simulink model "SiEngineController"  (R2024a)
settings: configuration reference "EngFixed10ms" (kept outside this file)
undefined symbols (not defined in the file): CtrlEcuTs, PlntEngAfrStoich
libraries: autolibengctrlr x1
settings Model: DataDictionary=VirtualDynoTemplate.sldd  ModifiedByFormat=The MathWorks, Inc.  Creator=The MathWorks, Inc.  LastModifiedBy=The MathWorks, Inc.
settings ConfigSetRef: SourceName=EngFixed10ms

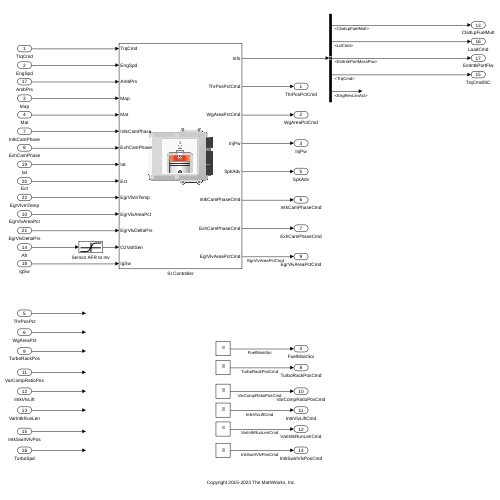
[thumbnail: Simulink's stored preview of the top-level diagram]
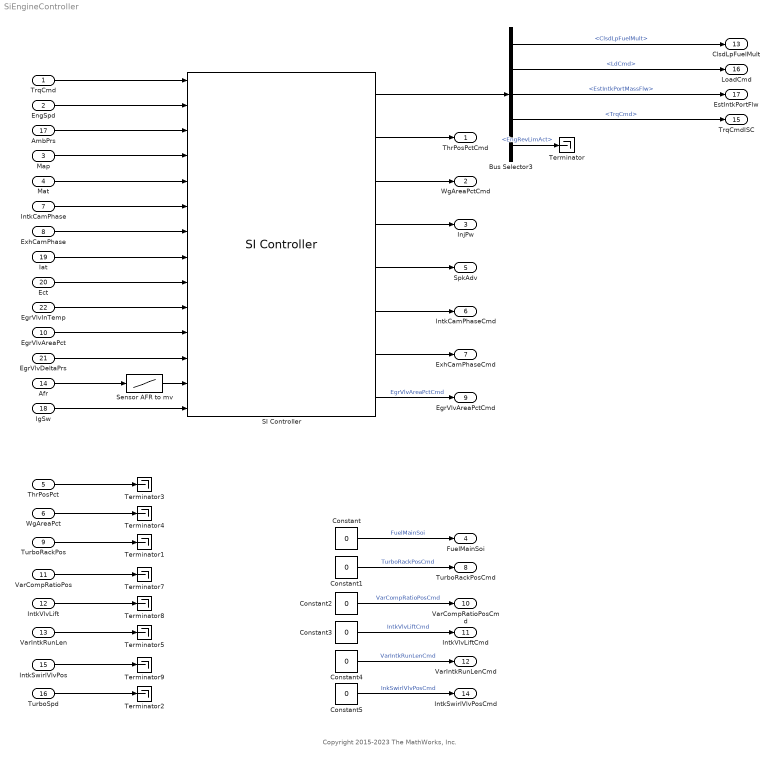
== system SiEngineController ==
  note: Copyright 2015-2023 The MathWorks, Inc.
  TrqCmd : Inport  OutDataTypeStr=double  Unit=N*m  PortDimensions=1
  EngSpd : Inport  Port=2  OutDataTypeStr=double  Unit=rpm  PortDimensions=1
  Map : Inport  Port=3  OutDataTypeStr=double  Unit=Pa  PortDimensions=1
  Mat : Inport  Port=4  OutDataTypeStr=double  Unit=K  PortDimensions=1
  ThrPosPct : Inport  Port=5  OutDataTypeStr=double  Unit=%  PortDimensions=1
  WgAreaPct : Inport  Port=6  OutDataTypeStr=double  Unit=%  PortDimensions=1
  IntkCamPhase : Inport  Port=7  OutDataTypeStr=double  Unit=deg  PortDimensions=1
  ExhCamPhase : Inport  Port=8  OutDataTypeStr=double  Unit=deg  PortDimensions=1
  TurboRackPos : Inport  Port=9  OutDataTypeStr=double  Unit=1  PortDimensions=1
  EgrVlvAreaPct : Inport  Port=10  OutDataTypeStr=double  Unit=%  PortDimensions=1
  VarCompRatioPos : Inport  Port=11  OutDataTypeStr=double  PortDimensions=1
  IntkVlvLift : Inport  Port=12  OutDataTypeStr=double  PortDimensions=1
  VarIntkRunLen : Inport  Port=13  OutDataTypeStr=double  PortDimensions=1
  Afr : Inport  Port=14  OutDataTypeStr=double  Unit=1  PortDimensions=1
  IntkSwirlVlvPos : Inport  Port=15  OutDataTypeStr=double  PortDimensions=1
  TurboSpd : Inport  Port=16  OutDataTypeStr=double  Unit=rpm  PortDimensions=1
  AmbPrs : Inport  Port=17  OutDataTypeStr=double  Unit=Pa  PortDimensions=1
  IgSw : Inport  Port=18  OutDataTypeStr=boolean  PortDimensions=1
  Iat : Inport  Port=19  OutDataTypeStr=double  Unit=K  PortDimensions=1
  Ect : Inport  Port=20  OutDataTypeStr=double  Unit=K  PortDimensions=1
  EgrVlvDeltaPrs : Inport  Port=21  OutDataTypeStr=double  Unit=Pa  PortDimensions=1
  EgrVlvInTemp : Inport  Port=22  OutDataTypeStr=double  Unit=K  PortDimensions=1
  Bus Selector3 : BusSelector  OutputSignals=ClsdLpFuelMult,LdCmd,EstIntkPortMassFlw,TrqCmd,EngRevLimAct
  Constant{,1..5} (6 alike) : Constant  Value=0  SampleTime=-1
  SI Controller : autolibengctrlr/SI Controller  AirEstOptionPopup=Dual Variable Cam Phasing  TrqEstOptionPopup=Torque Structure  f_lcmd=CtrlEcuLCmd  f_lcmd_tq_bpt=CtrlEcuLCmdTqBpt  f_lcmd_n_bpt=CtrlEcuLCmdSpdBpt  f_tap=CtrlEcuTap  f_tap_ld_bpt=CtrlEcuTapLBpt  f_tap_n_bpt=CtrlEcuTapNBpt  f_tpp=CtrlEcuTpp  f_tpp_tap_bpt=CtrlEcuTppTapBpt  f_wap=CtrlEcuWap  f_wap_ld_bpt=CtrlEcuWapLBpt  f_wap_n_bpt=CtrlEcuWapNBpt  f_icp=CtrlEcuIcp  f_ecp=CtrlEcuEcp  f_cp_ld_bpt=CtrlEcuCpLBpt  f_cp_n_bpt=CtrlEcuCpNBpt  f_egrpct_cmd=CtrlEcuEgrCmd  f_egrpct_ld_bpt=CtrlEcuEgrCmdLBpt  f_egrpct_n_bpt=CtrlEcuEgrCmdNBpt  f_egr_areapct_cmd=CtrlEcuEgrAreaCmd  f_egr_max_stdflow=CtrlEcuEgrMaxStdFlw  f_egr_areapct_nrmlzdflow_bpt=CtrlEcuEgrAreaNrmFlwBpt  f_egr_areapct_pr_bpt=CtrlEcuEgrAreaPrBpt  LambdaCmdOvrd=off  Sinj=PlntEngSinj  Nmin=1  afr_stoich=PlntEngAfrStoich  f_lamcmd=CtrlEcuLamCmd  f_lamcmd_ld_bpt=CtrlEcuLamCmdLBpt  f_lamcmd_n_bpt=CtrlEcuLamCmdNBpt  f_startup_lambda_delta=CtrlEcuStUpLamDelta  f_startup_lambda_delta_timecnst=CtrlEcuStUpLamDeltaTimeC  f_startup_ect_bpt=CtrlEcuStUpEctBpt  ClsdLpFuelEn=off  OpenLpDitherEn=off  LambdaDitherAmp=0.03  LambdaDitherFrq=0.75  ClsdLpFuelPGain=0.005  ClsdLpFuelIGain=0.05  ClsdLpFuelIntgLmt=0.2  O2ResetStoichVoltSen=2500  O2ResetMinVoltSen=0  O2ResetMaxVoltSen=5000  O2LearnUpdatePerSen=4  O2AmpMinVoltSen=250  O2ReadyVoltSen=1150  O2NotReadyVoltSen=1950  f_sa=CtrlEcuSa  f_sa_ld_bpt=CtrlEcuSaLBpt  f_sa_n_bpt=CtrlEcuSaNBpt  N_idle=CtrlEcuNidle  Trq_idlecmd_enable=1  Trq_idlecmd_max=50  Kp_idle=0.02  Ki_idle=0.01  EngRevLim=CtrlEcuRevLim  CrankSpeed=CtrlEcuCrkSpd  ESSEnable=on  ESSExternalPortEnable=off  EngStopTime=CtrlEcuStopTime  CatLightOffTime=CtrlEcuCatLOff  Ts=CtrlEcuTs  NCyl=PlntEngNCyl  Cps=PlntEngCps  Vd=PlntEngVd  Rair=EnvRair  Pstd=EnvAbsPrs  Tstd=EnvAirTemp  f_nv=PlntEngNv  f_nv_prs_bpt=PlntEngNvPrBpt  f_nv_n_bpt=PlntEngNvSpdBpt  f_vivc=PlntEngVivc  f_tm_corr_n_bpt=PlntEngTmCorrNBpt  f_vivc_icp_bpt=PlntEngVivcBpt  f_tm_corr=PlntEngTmCorr  f_tm_corr_nd_bpt=PlntEngTmCorrNdBpt  f_mdot_intk=CtrlEngMdotIntk  f_mdot_intk_ecp_bpt=PlntEngMdotIntkEcpBpt  f_mdot_trpd_bpt=PlntEngMdotTrpdBpt  f_mdot_air_corr=PlntEngMdotAirCorr  f_mdot_air_corr_ld_bpt=PlntEngMdotAirCorrLdBpt  f_mdot_air_n_bpt=PlntEngMdotAirCorrNBpt  tau_egr=CtrlEcuEgrTau  f_intksys_stdflow_pr=CtrlEcuInkStdFlwPr  f_intksys_stdflow_bpt=CtrlEcuInkStdFlwBpt  f_egr_stdflow=CtrlEcuEgrStdFlw  f_egr_stdflow_pr_bpt=CtrlEcuEgrStdFlwPrBpt  f_egr_stdflow_egrap_bpt=CtrlEcuEgrStdFlwEgrApBpt  f_tq_nl=PlntEngTqTbl  f_tq_nl_l_bpt=PlntEngTqTblLBpt  f_tq_nl_n_bpt=PlntEngTqTblNBpt  f_tq_inr=CtrlEngInTrqMap  f_tq_fric=CtrlEngTqFric  f_fric_temp_mod=PlntEngFricTMod  f_fric_temp_bpt=PlntEngFricTBpt  f_tq_pump=CtrlEngTqPump  f_sa_opt=CtrlEngSAOpt  f_tq_inr_l_bpt=CtrlEngInTrqLdBpt  f_tq_inr_n_bpt=CtrlEngInTrqSpdBpt  f_m_sa=PlntEngMSa  f_del_sa_bpt=PlntEngDelSaBpt  f_m_lam=PlntEngMLam  f_m_lam_bpt=PlntEngMLamBpt  f_t_exh=PlntEngTexh  f_t_exh_l_bpt=PlntEngTexhLBpt  f_t_exh_n_bpt=PlntEngTexhNBpt
  Sensor AFR to mv : Lookup  InputValues="PlntEngAfrStoich+[-0.1460         0    0.1460]"  Table="[950   450    50]"  LookUpMeth=Interpolation-Use End Values  SaturateOnIntegerOverflow=off
  Terminator{,1..5,7..9} (9 alike) : Terminator
  ThrPosPctCmd : Outport  OutDataTypeStr=double  Unit=%  PortDimensions=1  VectorParamsAs1DForOutWhenUnconnected=off
  WgAreaPctCmd : Outport  Port=2  OutDataTypeStr=double  Unit=%  PortDimensions=1  VectorParamsAs1DForOutWhenUnconnected=off
  InjPw : Outport  Port=3  OutDataTypeStr=double  Unit=ms  PortDimensions=1  VectorParamsAs1DForOutWhenUnconnected=off
  FuelMainSoi : Outport  Port=4  OutDataTypeStr=double  Unit=deg  PortDimensions=1  VectorParamsAs1DForOutWhenUnconnected=off
  SpkAdv : Outport  Port=5  OutDataTypeStr=double  Unit=deg  PortDimensions=1  VectorParamsAs1DForOutWhenUnconnected=off
  IntkCamPhaseCmd : Outport  Port=6  OutDataTypeStr=double  Unit=deg  PortDimensions=1  VectorParamsAs1DForOutWhenUnconnected=off
  ExhCamPhaseCmd : Outport  Port=7  OutDataTypeStr=double  Unit=deg  PortDimensions=1  VectorParamsAs1DForOutWhenUnconnected=off
  TurboRackPosCmd : Outport  Port=8  OutDataTypeStr=double  Unit=1  PortDimensions=1  VectorParamsAs1DForOutWhenUnconnected=off
  EgrVlvAreaPctCmd : Outport  Port=9  OutDataTypeStr=double  Unit=%  PortDimensions=1  VectorParamsAs1DForOutWhenUnconnected=off
  VarCompRatioPosCmd : Outport  Port=10  OutDataTypeStr=double  PortDimensions=1  VectorParamsAs1DForOutWhenUnconnected=off
  IntkVlvLiftCmd : Outport  Port=11  OutDataTypeStr=double  PortDimensions=1  VectorParamsAs1DForOutWhenUnconnected=off
  VarIntkRunLenCmd : Outport  Port=12  OutDataTypeStr=double  PortDimensions=1  VectorParamsAs1DForOutWhenUnconnected=off
  ClsdLpFuelMult : Outport  Port=13  OutDataTypeStr=double  Unit=1  PortDimensions=1  VectorParamsAs1DForOutWhenUnconnected=off
  IntkSwirlVlvPosCmd : Outport  Port=14  OutDataTypeStr=double  PortDimensions=1  VectorParamsAs1DForOutWhenUnconnected=off
  TrqCmdISC : Outport  Port=15  OutDataTypeStr=double  Unit=N*m  PortDimensions=1  VectorParamsAs1DForOutWhenUnconnected=off
  LoadCmd : Outport  Port=16  OutDataTypeStr=double  Unit=1  PortDimensions=1  VectorParamsAs1DForOutWhenUnconnected=off
  EstIntkPortFlw : Outport  Port=17  OutDataTypeStr=double  Unit=kg/s  PortDimensions=1  VectorParamsAs1DForOutWhenUnconnected=off
  wires:
  AmbPrs/1 -> SI Controller/3
  Map/1 -> SI Controller/4
  Mat/1 -> SI Controller/5
  IntkCamPhase/1 -> SI Controller/6
  ExhCamPhase/1 -> SI Controller/7
  SI Controller/1 -> Bus Selector3/1
  Bus Selector3/4 -> TrqCmdISC/1  "<TrqCmd>"
  Constant1/1 -> TurboRackPosCmd/1  "TurboRackPosCmd"
  EngSpd/1 -> SI Controller/2
  TrqCmd/1 -> SI Controller/1
  Bus Selector3/3 -> EstIntkPortFlw/1  "<EstIntkPortMassFlw>"
  Bus Selector3/2 -> LoadCmd/1  "<LdCmd>"
  Constant/1 -> FuelMainSoi/1  "FuelMainSoi"
  TurboRackPos/1 -> Terminator1/1
  TurboSpd/1 -> Terminator2/1
  SI Controller/4 -> InjPw/1
  IntkSwirlVlvPos/1 -> Terminator9/1
  VarIntkRunLen/1 -> Terminator5/1
  IntkVlvLift/1 -> Terminator8/1
  VarCompRatioPos/1 -> Terminator7/1
  Constant5/1 -> IntkSwirlVlvPosCmd/1  "InkSwirlVlvPosCmd"
  Constant4/1 -> VarIntkRunLenCmd/1  "VarIntkRunLenCmd"
  Constant3/1 -> IntkVlvLiftCmd/1  "IntkVlvLiftCmd"
  Constant2/1 -> VarCompRatioPosCmd/1  "VarCompRatioPosCmd"
  ThrPosPct/1 -> Terminator3/1
  WgAreaPct/1 -> Terminator4/1
  SI Controller/6 -> IntkCamPhaseCmd/1
  SI Controller/7 -> ExhCamPhaseCmd/1
  SI Controller/5 -> SpkAdv/1
  SI Controller/2 -> ThrPosPctCmd/1
  SI Controller/3 -> WgAreaPctCmd/1
  SI Controller/8 -> EgrVlvAreaPctCmd/1  "EgrVlvAreaPctCmd"
  EgrVlvAreaPct/1 -> SI Controller/11
  EgrVlvDeltaPrs/1 -> SI Controller/12
  Iat/1 -> SI Controller/8
  EgrVlvInTemp/1 -> SI Controller/10
  Ect/1 -> SI Controller/9
  Bus Selector3/5 -> Terminator/1  "<EngRevLimAct>"
  Sensor AFR to mv/1 -> SI Controller/13
  Afr/1 -> Sensor AFR to mv/1
  Bus Selector3/1 -> ClsdLpFuelMult/1  "<ClsdLpFuelMult>"
  IgSw/1 -> SI Controller/14
